simulink model "drone"  (R2024b)
settings: Solver=VariableStepAuto  StartTime=0.0  StopTime=Tfinal  RelTol=1e-3
values from neighbouring files (symbols this model uses):
  A = [0 0 0 0 0 0 1 0 0 0 0 0 ... (first row only)    [SetDroneControl.m]    (also in dron.m)
  At = As-Fs*Kb    [SetDroneControl.m]    (also in dron.m)
  B = [0   0    0    0 ... (first row only)    [SetDroneControl.m]    (also in dron.m)
  Bt = Bs-Fs*(Ka+Kb*Ke)    [SetDroneControl.m]    (also in dron.m)
  C = eye(12)    [SetDroneControl.m]    (also in dron.m)
  Ct = -Kb    [SetDroneControl.m]    (also in dron.m)
  D = zeros(12,4)    [SetDroneControl.m]    (also in dron.m)
  Dt = -(Ka+Kb*Ke)    [SetDroneControl.m]    (also in dron.m)
  IC = [0 ... (first row only)    [SetDroneControl.m]    (also in dron.m)
  positionTolerance = 0.1    [SetDroneControl.m]
  ts = 0.01    [SetDroneControl.m]
  WayPts = [wayPoints, timeForWaypointPasage']    [XYZsignal.m]
undefined symbols (not defined in the file or in its folder): den1, num1
settings Model: Creator=annab  LastModifiedBy=oggys

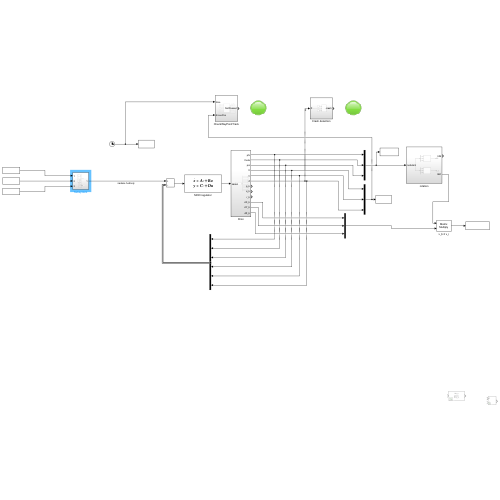
[thumbnail: Simulink's stored preview of the top-level diagram]
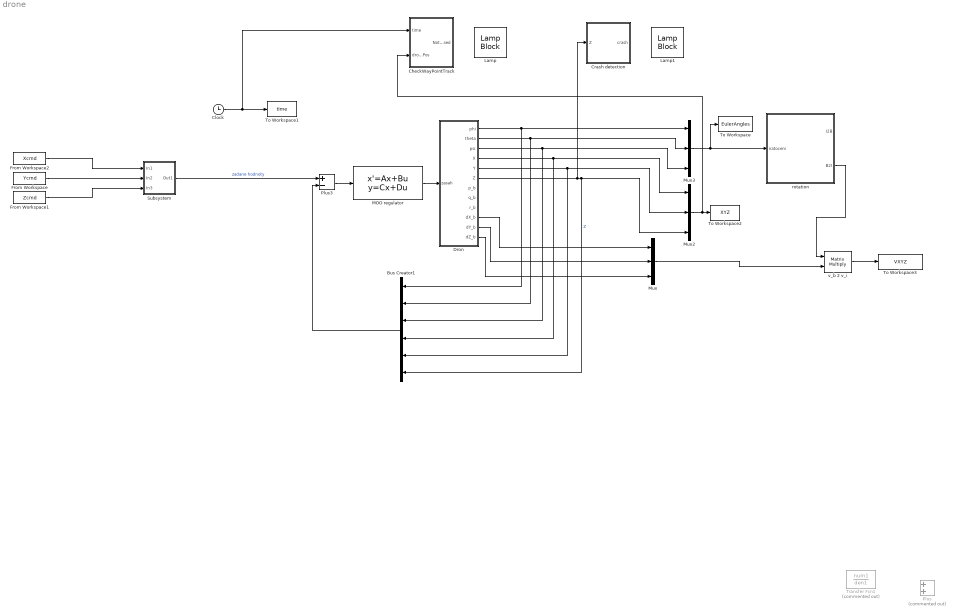
== system drone ==
  Bus Creator1 : BusCreator  Inputs=6
  CheckWayPointTrack : Subsystem
  Clock : Clock
  Crash detection : Subsystem
  Dron : Subsystem
  From Workspace : FromWorkspace  VariableName=Ycmd  SampleTime=ts
  From Workspace1 : FromWorkspace  VariableName=Zcmd  SampleTime=ts
  From Workspace2 : FromWorkspace  VariableName=Xcmd  SampleTime=ts
  Lamp : LampBlock  LabelPosition=Hide
  Lamp1 : LampBlock  LabelPosition=Hide
  MOO regulator : StateSpace  A=At  B=Bt  C=-Ct  D=-Dt  InitialCondition=0
  Mux : Mux  Inputs=3
  Mux2 : Mux  Inputs=3
  Mux3 : Mux  Inputs=3
  Plus : Sum  Commented=on
  Plus3 : Sum  Inputs=+-
  Subsystem : Subsystem
  To Workspace : ToWorkspace  VariableName=EulerAngles  SampleTime=ts
  To Workspace1 : ToWorkspace  VariableName=time  SampleTime=ts
  To Workspace2 : ToWorkspace  VariableName=XYZ  SampleTime=ts
  To Workspace3 : ToWorkspace  VariableName=VXYZ  SampleTime=ts
  Transfer Fcn1 : TransferFcn  Commented=on  Numerator=num1  Denominator=den1
  rotation : Subsystem
  v_b 2 v_i : Product  Multiplication=Matrix(*)
  wires:
  Clock/1 -> CheckWayPointTrack/1(time), To Workspace1/1
  Plus3/1 -> MOO regulator/1
  Bus Creator1/1 -> Plus3/2
  Mux2/1 -> CheckWayPointTrack/2(dronePos), To Workspace2/1
  Dron/2(theta) -> Mux3/2, Bus Creator1/2
  Dron/1(phi) -> Mux3/1, Bus Creator1/1
  Dron/4(X) -> Mux2/1, Bus Creator1/4
  Dron/3(psi) -> Mux3/3, Bus Creator1/3
  Dron/5(Y) -> Mux2/2, Bus Creator1/5
  MOO regulator/1 -> Dron/1(zasah)
  From Workspace2/1 -> Subsystem/1(In1)
  From Workspace/1 -> Subsystem/2(In2)
  From Workspace1/1 -> Subsystem/3(In3)
  Subsystem/1(Out1) -> Plus3/1  "zadane hodnoty"
  Dron/10(dX_b) -> Mux/1
  Dron/11(dY_b) -> Mux/2
  Dron/12(dZ_b) -> Mux/3
  rotation/2(B2I) -> v_b 2 v_i/1
  Mux/1 -> v_b 2 v_i/2
  v_b 2 v_i/1 -> To Workspace3/1
  Mux3/1 -> To Workspace/1, rotation/1(natoceni)
  Dron/6(Z) -> Mux2/3, Bus Creator1/6, Crash detection/1(Z)  "Z"

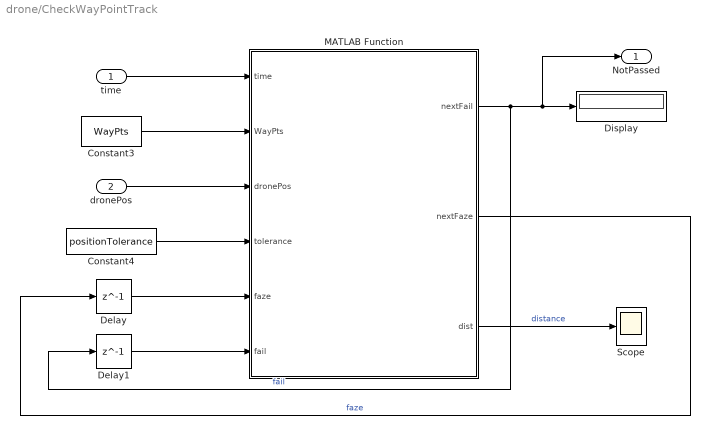
== system drone/CheckWayPointTrack ==
  time : Inport
  dronePos : Inport  Port=2
  Constant3 : Constant  Value=WayPts
  Constant4 : Constant  Value=positionTolerance
  Delay : Delay  DelayLength=1  InitialCondition=1
  Delay1 : Delay  DelayLength=1  InitialCondition=0
  Display : Display
  MATLAB Function : MATLAB Function  TreatAsAtomicUnit=on
  Scope : Scope
  NotPassed : Outport
  wires:
  Delay/1 -> MATLAB Function/5(faze)
  MATLAB Function/1(nextFail) -> NotPassed/1, Display/1, Delay1/1  "fail"
  Constant4/1 -> MATLAB Function/4(tolerance)
  MATLAB Function/3(dist) -> Scope/1  "distance"
  Delay1/1 -> MATLAB Function/6(fail)
  MATLAB Function/2(nextFaze) -> Delay/1  "faze"
  Constant3/1 -> MATLAB Function/2(WayPts)
  dronePos/1 -> MATLAB Function/3(dronePos)
  time/1 -> MATLAB Function/1(time)

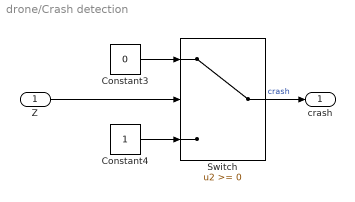
== system drone/Crash detection ==
  Z : Inport
  Constant3 : Constant  Value=0
  Constant4 : Constant
  Switch : Switch  SaturateOnIntegerOverflow=off  InputSameDT=off
  crash : Outport
  wires:
  Z/1 -> Switch/2
  Switch/1 -> crash/1  "crash"
  Constant3/1 -> Switch/1
  Constant4/1 -> Switch/3

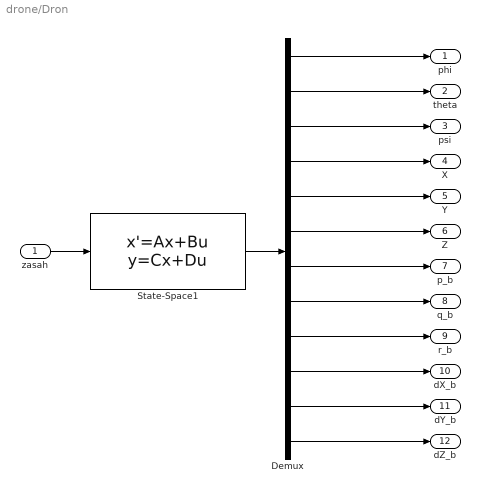
== system drone/Dron ==
  zasah : Inport
  Demux : Demux  Outputs=12
  State-Space1 : StateSpace  A=A  B=B  C=C  D=D  InitialCondition=IC
  phi : Outport
  theta : Outport  Port=2
  psi : Outport  Port=3
  X : Outport  Port=4
  Y : Outport  Port=5
  Z : Outport  Port=6
  p_b : Outport  Port=7
  q_b : Outport  Port=8
  r_b : Outport  Port=9
  dX_b : Outport  Port=10
  dY_b : Outport  Port=11
  dZ_b : Outport  Port=12
  wires:
  zasah/1 -> State-Space1/1
  State-Space1/1 -> Demux/1
  Demux/4 -> X/1
  Demux/3 -> psi/1
  Demux/2 -> theta/1
  Demux/1 -> phi/1
  Demux/10 -> dX_b/1
  Demux/6 -> Z/1
  Demux/9 -> r_b/1
  Demux/5 -> Y/1
  Demux/11 -> dY_b/1
  Demux/7 -> p_b/1
  Demux/12 -> dZ_b/1
  Demux/8 -> q_b/1

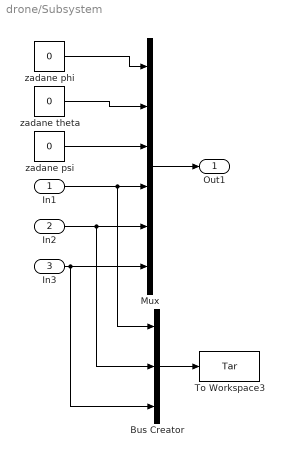
== system drone/Subsystem ==
  In1 : Inport
  In2 : Inport  Port=2
  In3 : Inport  Port=3
  Bus Creator : BusCreator  Inputs=3
  Mux : Mux  Inputs=6
  To Workspace3 : ToWorkspace  VariableName=Tar  SampleTime=ts
  zadane phi : Constant  Value=0
  zadane psi : Constant  Value=0
  zadane theta : Constant  Value=0
  Out1 : Outport
  wires:
  zadane psi/1 -> Mux/3
  zadane phi/1 -> Mux/1
  zadane theta/1 -> Mux/2
  In3/1 -> Bus Creator/3, Mux/6
  In1/1 -> Mux/4, Bus Creator/1
  Mux/1 -> Out1/1
  In2/1 -> Bus Creator/2, Mux/5
  Bus Creator/1 -> To Workspace3/1

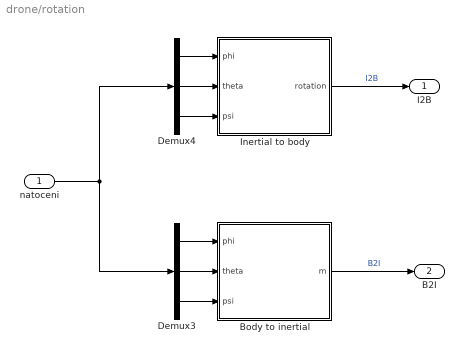
== system drone/rotation ==
  natoceni : Inport
  Body to inertial : MATLAB Function  TreatAsAtomicUnit=on
  Demux3 : Demux  Outputs=3
  Demux4 : Demux  Outputs=3
  Inertial to body : MATLAB Function  TreatAsAtomicUnit=on
  I2B : Outport
  B2I : Outport  Port=2
  wires:
  Demux4/2 -> Inertial to body/2(theta)
  Demux3/1 -> Body to inertial/1(phi)
  Body to inertial/1(m) -> B2I/1  "B2I"
  natoceni/1 -> Demux4/1, Demux3/1
  Demux4/3 -> Inertial to body/3(psi)
  Demux4/1 -> Inertial to body/1(phi)
  Demux3/2 -> Body to inertial/2(theta)
  Demux3/3 -> Body to inertial/3(psi)
  Inertial to body/1(rotation) -> I2B/1  "I2B"

== matlab function drone/rotation/Body to inertial ==
  data: phi input; m output; theta input; psi input
function m = fcn(phi,theta,psi)
    T_BtoV2 = [
                [1 0 0];
                [0 cos(-phi) sin(-phi)];
                [0 -sin(-phi) cos(-phi)]
              ];
    T_V2toV1 = [
                [cos(-theta) 0 -sin(-theta)];
                [0 1 0];
                [sin(-theta) 0 cos(-theta)]
               ];
    T_V1toI = [
                [cos(-psi) sin(-psi) 0];
                [-sin(-psi) cos(-psi) 0];
                [0 0 1]
              ];

    m = T_V1toI * T_V2toV1 * T_BtoV2;

== matlab function drone/CheckWayPointTrack/MATLAB Function ==
  data: time input; nextFail output; WayPts input; dronePos input; tolerance input; faze input; fail input; nextFaze output; dist output
function [nextFail, nextFaze, dist] = check_waypoints(time, WayPts, dronePos, tolerance, faze, fail)

    nextFail = fail;
    nextFaze = faze;
    dist = 0;

    if faze > size(WayPts,1)
        return
    end
    criticalTime = WayPts(faze,4);
    dist = abs(norm(WayPts(faze,1:3)) - norm(dronePos));
    if dist <= tolerance
        nextFaze = faze + 1;
    else 
        nextFaze = faze;
    end

    if fail == 1
        nextFail = 1;
        return
    end

    if time > criticalTime
        nextFail = 1;
    else
        nextFail = 0;
    end
end

== matlab function drone/rotation/Inertial to body ==
  data: phi input; rotation output; theta input; psi input
function rotation = RollPitchYaw2Rotation(phi,theta,psi)

    % Rotation matrices
    R3 = [cos(psi) sin(psi) 0;...
          -sin(psi) cos(psi) 0;...
          0 0 1];
    R2 = [cos(theta) 0 -sin(theta);...
          0 1 0;...
          sin(theta) 0 cos(theta)];
    R1 = [1 0 0;...
          0 cos(phi) sin(phi);...
          0 -sin(phi) cos(phi)];
    
    % Rotation
    rotation = R1 * R2 * R3; 
end
